simulink model "modelisation"  (R2024b)
settings: Solver=VariableStepAuto  StartTime=0.0  StopTime=10.0  RelTol=1e-3
model workspace (MAT data in the model file):
  B_c = 1
  B_m = 1
  J_c = 1
  J_m = 1
  K_bb = 1
  K_m = 1
  K_t = 1
  L_m = 1
  N = 1
  R_m = 1
  V_m = 1000
  n_m = 1
settings Model: Creator=thoma  LastModifiedBy=zpoul

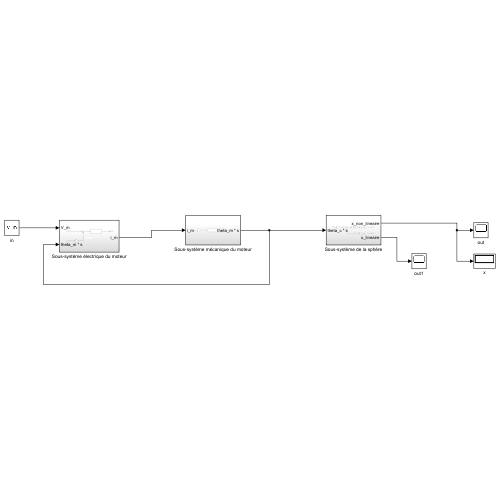
[thumbnail: Simulink's stored preview of the top-level diagram]
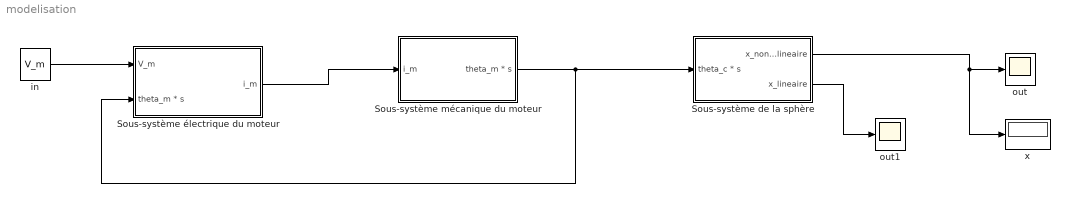
== system modelisation ==
  Sous-système de la sphère : Subsystem
  Sous-système mécanique du moteur : Subsystem
  Sous-système électrique du moteur : Subsystem
  in : Constant  Value=V_m
  out : Scope
  out1 : Scope
  x : Display
  wires:
  in/1 -> Sous-système électrique du moteur/1(V_m)
  Sous-système électrique du moteur/1(i_m) -> Sous-système mécanique du moteur/1(i_m)
  Sous-système mécanique du moteur/1(theta_m * s) -> Sous-système de la sphère/1(theta_c * s), Sous-système électrique du moteur/2(theta_m * s)
  Sous-système de la sphère/1(x_non_lineaire) -> x/1, out/1
  Sous-système de la sphère/2(x_lineaire) -> out1/1

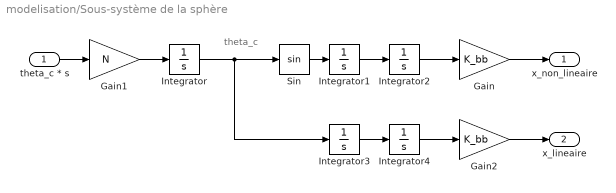
== system modelisation/Sous-système de la sphère ==
  note: theta_c
  theta_c * s : Inport
  Gain : Gain  Gain=K_bb
  Gain1 : Gain  Gain=N
  Gain2 : Gain  Gain=K_bb
  Integrator{,1..4} (5 alike) : Integrator
  Sin : Trigonometry
  x_non_lineaire : Outport
  x_lineaire : Outport  Port=2
  wires:
  Sin/1 -> Integrator1/1
  Integrator1/1 -> Integrator2/1
  Integrator2/1 -> Gain/1
  Gain/1 -> x_non_lineaire/1
  theta_c * s/1 -> Gain1/1
  Gain1/1 -> Integrator/1
  Integrator3/1 -> Integrator4/1
  Gain2/1 -> x_lineaire/1
  Integrator/1 -> Integrator3/1, Sin/1
  Integrator4/1 -> Gain2/1

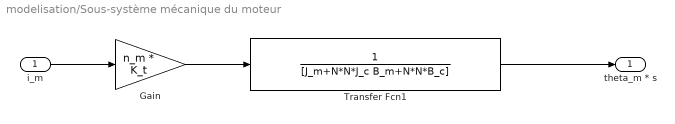
== system modelisation/Sous-système mécanique du moteur ==
  i_m : Inport
  Gain : Gain  Gain=n_m * K_t
  Transfer Fcn1 : TransferFcn  Denominator=[J_m+N*N*J_c B_m+N*N*B_c]
  theta_m * s : Outport
  wires:
  i_m/1 -> Gain/1
  Transfer Fcn1/1 -> theta_m * s/1
  Gain/1 -> Transfer Fcn1/1

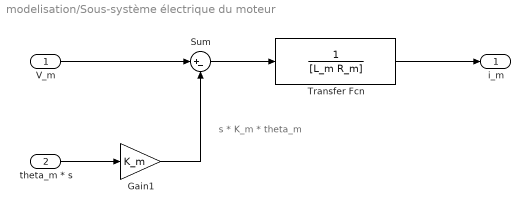
== system modelisation/Sous-système électrique du moteur ==
  note: s * K_m * theta_m
  V_m : Inport
  theta_m * s : Inport  Port=2
  Gain1 : Gain  Gain=K_m
  Sum : Sum  Inputs=|+-
  Transfer Fcn : TransferFcn  Denominator=[L_m R_m]
  i_m : Outport
  wires:
  V_m/1 -> Sum/1
  theta_m * s/1 -> Gain1/1
  Sum/1 -> Transfer Fcn/1
  Transfer Fcn/1 -> i_m/1
  Gain1/1 -> Sum/2
